simulink model "E1b"  (R2017a)
settings: Solver=ode3  StartTime=0.0  StopTime=100.0  FixedStep=0.01  RelTol=1e-3
undefined symbols (not defined in the file): Discrete, Time
libraries: ctrlSharedLib x1
settings Model: Creator=Soutrik  LastModifiedBy=Soutrik

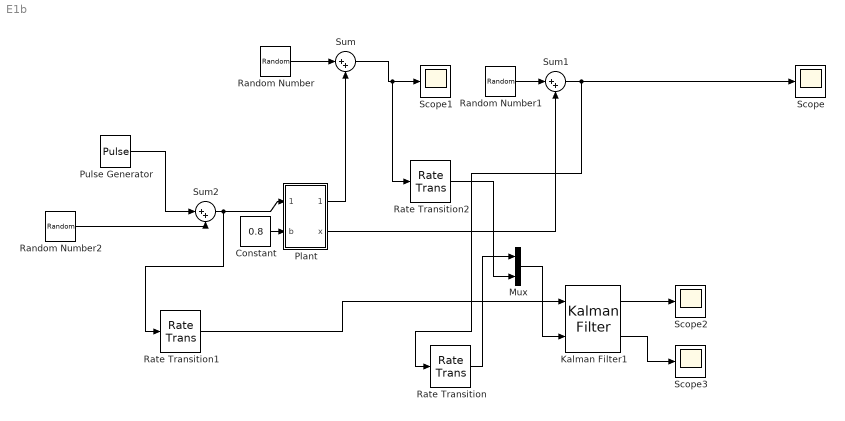
== system E1b ==
  Constant : Constant  Value=0.8
  Kalman Filter1 : ctrlSharedLib/Kalman Filter  TimeDomain=Discrete-Time  UseCurrentEstimator=on  ModelSource=Individual A, B, C, D matrices  ModelSourceVariable=ss(0.95,1,1,0,1)  A=[0 1;-1 -0.8]  B=[0;1]  C=[1 0]  D=0  NumberOfStates=2  NumberOfInputs=1  NumberOfOutputs=1  InitialEstimateSource=Dialog  X0=0  P0=10  UseK=off  UseGH=on  NumberOfProcessNoiseInputs=1  G=[1 0;0 1]  TimeInvariantG=on  H=0  TimeInvariantH=on  Q=0.05  TimeInvariantQ=on  R=1  TimeInvariantR=on  N=0  TimeInvariantN=on  AddInputPort=on  AddEnablePort=off  OutputEstimatedY=off  OutputP=on  Ts=1
  Mux : Mux  Inputs=2
  Plant : Subsystem
  Pulse Generator : DiscretePulseGenerator  PulseType=Time based  Period=10  PulseWidth=50
  Random Number : RandomNumber  Variance=0.001  Seed=47  SampleTime=0.1
  Random Number1 : RandomNumber  Variance=0.001  Seed=89  SampleTime=0.1
  Random Number2 : RandomNumber  Variance=0.001  Seed=59  SampleTime=0.1
  Rate Transition : RateTransition
  Rate Transition1 : RateTransition
  Rate Transition2 : RateTransition
  Scope{,1..3} (4 alike) : Scope
  Sum : Sum  Inputs=|++
  Sum1 : Sum  Inputs=|++
  Sum2 : Sum  Inputs=|++
  wires:
  Random Number/1 -> Sum/1
  Sum/1 -> Rate Transition2/1, Scope1/1
  Random Number1/1 -> Sum1/1
  Plant/1(xdot) -> Sum/2
  Plant/2(x) -> Sum1/2
  Random Number2/1 -> Sum2/2
  Pulse Generator/1 -> Sum2/1
  Constant/1 -> Plant/2(b)
  Sum2/1 -> Plant/1(In1), Rate Transition1/1
  Sum1/1 -> Rate Transition/1, Scope/1
  Rate Transition1/1 -> Kalman Filter1/1
  Kalman Filter1/1 -> Scope2/1
  Kalman Filter1/2 -> Scope3/1
  Rate Transition2/1 -> Mux/2
  Rate Transition/1 -> Mux/1
  Mux/1 -> Kalman Filter1/2

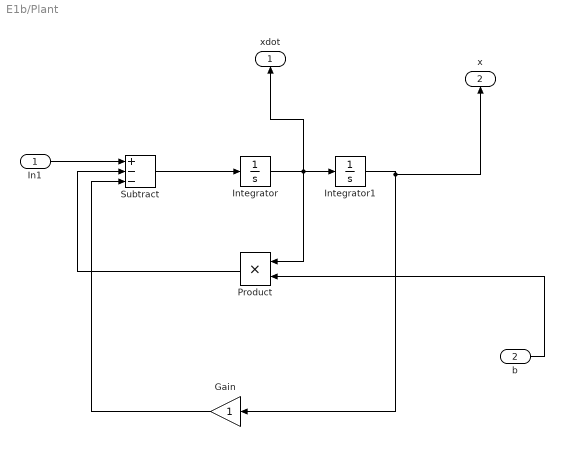
== system E1b/Plant ==
  In1 : Inport
  b : Inport  Port=2
  Gain : Gain
  Integrator : Integrator
  Integrator1 : Integrator
  Product : Product
  Subtract : Sum  Inputs=+--
  xdot : Outport
  x : Outport  Port=2
  wires:
  Product/1 -> Subtract/2
  Subtract/1 -> Integrator/1
  Gain/1 -> Subtract/3
  In1/1 -> Subtract/1
  Integrator/1 -> xdot/1, Product/1, Integrator1/1
  Integrator1/1 -> x/1, Gain/1
  b/1 -> Product/2
